simulink model "Loops9"  (Simulink 6.0)
settings: Solver=ode45  StartTime=0.0  StopTime=10.0  RelTol=1e-3
settings Model: Creator=scaife  LastModifiedBy=scaife  ExtModeAutoUpdateStatusClock=off
settings DataIOCC: SignalLoggingName=sigsOut
settings DebuggingCC: SolverPrmCheckMsg=none
settings HardwareCC: TargetUnknown=on
settings GRTTargetCC: ModelReferenceCompliant=off  MatFileLogging=off

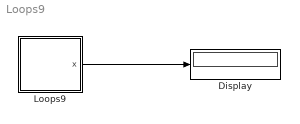
== system Loops9 ==
  Display : Display
  Loops9 : Stateflow chart
  wires:
  Loops9/1(x) -> Display/1

== stateflow chart Loops9 ==
  state A
  state B
  (default) -> A
  (junction 6) -> B : [x==0]
  (junction 6) -> (junction 5) : [x==1]
  A -> (junction 5) : {x=0}
  (junction 5) -> (junction 6) : [x==0]
  B -> (junction 6) : {x=1}
  (junction 5) -> A : [x==1]
  data: x output int32
